simulink library "RfftLib"  (R2022b)
settings: Solver=VariableStepAuto  StartTime=0.0  StopTime=10.0  RelTol=1e-3
libraries: HandyTextFile x7, ITC x2, $bdroot x2
settings Model: Creator=ud1041536  LastModifiedBy=fz1054048
settings SolverCC: AlgebraicLoopSolver=TrustRegion
settings DebuggingCC: UnconnectedInputMsg=warning  UnconnectedOutputMsg=warning  UnconnectedLineMsg=warning  SFMachineParentedDataDiag=warning  ArithmeticOperatorsInVariantConditions=warning
settings ModelReferenceCC: EnableRefExpFcnMdlSchedulingChecks=on
settings SFSimCC: CustomCodeUndefinedFunction=UseInterfaceOnly
settings RTWCC: DLArmComputeVersion=19.05

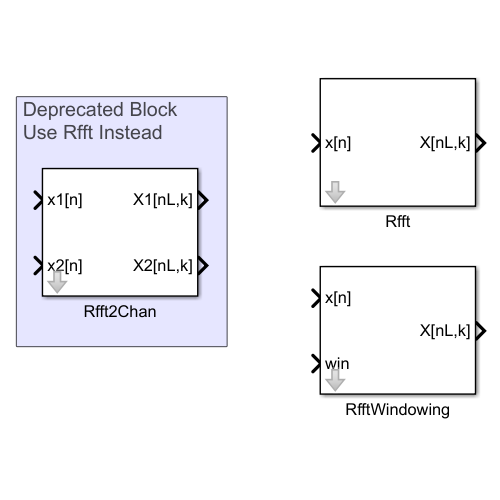
[thumbnail: Simulink's stored preview of the top-level diagram]
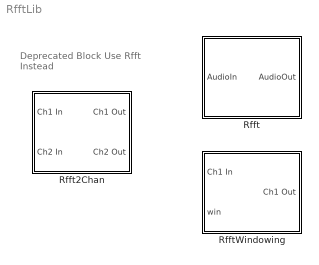
== system RfftLib ==
  note: Deprecated Block
      | Use Rfft Instead
  Rfft : Subsystem  Description=This block computes the Fourier Transform using an optimized FFT for real 2-channel input.  mask(Blocklib Rfft){Config=[]}
      mask prompts: Config "RfftConfig"
      mask help:
      | See 'Help' or run
      | >> help RfftConfig
      mask init:
      | blkh=gcbh;
      | Config=BTConfig.Assert(blkh,Config);
      | 
      | Config.Validate();
      | Config.DoMaskInit(blkh);
      mask Help: eval('help RfftConfig')
      mask Display:
      | port_label('input',1,'x[n]')
      | port_label('output',1,'X[nL,k]')
  Rfft2Chan : Subsystem  Description=This block computes the Fourier Transform using an optimized FFT for real 2-channel input.  mask(Blocklib Rfft2Chan){Config=[]}
      mask prompts: Config "Rfft2ChanConfig"
      mask help:
      | See 'Help' or run
      | >> help Rfft2ChanConfig
      mask init:
      | blkh=gcbh;
      | 
      | Config=BTConfig.Assert(blkh,Config);
      | 
      | Config.Validate();
      | Config.DoMaskInit(blkh);
      mask Help: eval('help Rfft2ChanConfig')
      mask Display:
      | port_label('input',1,'x1[n]')
      | port_label('input',2,'x2[n]')
      | port_label('output',1,'X1[nL,k]')
      | port_label('output',2,'X2[nL,k]')
  RfftWindowing : Subsystem  Description=This block computes the Fourier Transform using an optimized FFT for real 2-channel input.  mask(Blocklib RfftWindowing){Config=[]}
      mask prompts: Config "RfftWindowingConfig"
      mask help:
      | See 'Help' or run
      | >> help RfftWindowingConfig
      mask init:
      | blkh=gcbh;
      | Config=BTConfig.Assert(blkh,Config);
      | 
      | Config.Validate();
      | Config.DoMaskInit(blkh);
      mask Help: eval('help RfftWindowingConfig')
      mask Display:
      | port_label('input',1,'x[n]')
      | port_label('input',2,'win')
      | port_label('output',1,'X[nL,k]')

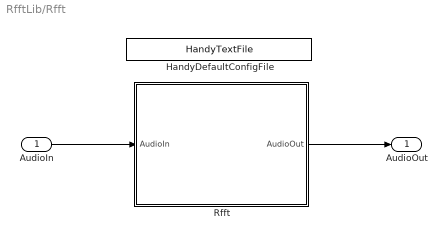
== system RfftLib/Rfft ==
  AudioIn : Inport
  HandyDefaultConfigFile : HandyTextFile/HandyTextFile  TemplateSource=Config  FileSuffix=Init  OpenDialogOnLoad=off  UseThisBlockName=off  AddGrandParentNamePrefix=off  TheDefaultText=|  ShowInLibBrowser=on
      | % $(FILENAME) Setup model parameters for each "Init" callback (e.g. update diagram)
      | sample_rate_in_hertz = 44100;
      | frame_size = 32;
      | sysin_channel_count = 2;
      settings: SourceProductName=Bose Talaria
  Rfft : Subsystem  Variant=on  VariantControl=Choice
  AudioOut : Outport  VectorParamsAs1DForOutWhenUnconnected=off
      settings: SignalType=complex
  wires:
  Rfft/1(AudioOut) -> AudioOut/1
  AudioIn/1 -> Rfft/1(AudioIn)

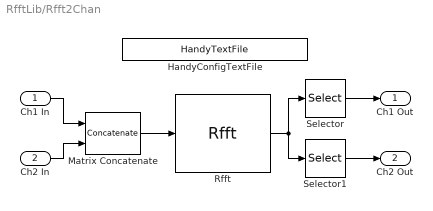
== system RfftLib/Rfft2Chan ==
  Ch1 In : Inport
  Ch2 In : Inport  Port=2
  HandyConfigTextFile : HandyTextFile/HandyTextFile  TemplateSource=Config  FileSuffix=File  OpenDialogOnLoad=off  UseThisBlockName=off  AddGrandParentNamePrefix=off  TheDefaultText=% $(FILENAME) $(PREFIX) $(SUFFIX)  ShowInLibBrowser=on
      settings: SourceProductName=Bose Talaria
  Matrix Concatenate : Concatenate  Mode=Multidimensional array  ConcatenateDimension=2
  Rfft : $bdroot/Rfft  Description=This block computes the Fourier Transform using an optimized FFT for real 2-channel input.  Config=Config
  Selector : Selector  NumberOfDimensions=2  InputPortWidth=3  IndexOptions=Select all,Index vector (dialog)  Indices=[1 3],1  OutputSizes=1,1
  Selector1 : Selector  NumberOfDimensions=2  InputPortWidth=3  IndexOptions=Select all,Index vector (dialog)  Indices=[1 3],2  OutputSizes=1,1
  Ch1 Out : Outport  VectorParamsAs1DForOutWhenUnconnected=off
  Ch2 Out : Outport  Port=2  VectorParamsAs1DForOutWhenUnconnected=off
  wires:
  Ch1 In/1 -> Matrix Concatenate/1
  Ch2 In/1 -> Matrix Concatenate/2
  Matrix Concatenate/1 -> Rfft/1
  Selector/1 -> Ch1 Out/1
  Rfft/1 -> Selector1/1, Selector/1
  Selector1/1 -> Ch2 Out/1

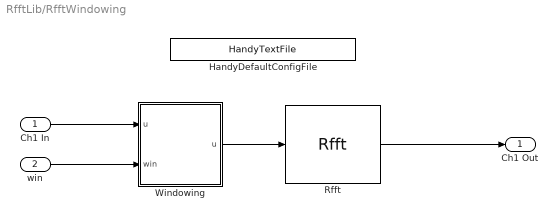
== system RfftLib/RfftWindowing ==
  Ch1 In : Inport
  win : Inport  Port=2
  HandyDefaultConfigFile : HandyTextFile/HandyTextFile  TemplateSource=Config  FileSuffix=Init  OpenDialogOnLoad=off  UseThisBlockName=off  AddGrandParentNamePrefix=off  TheDefaultText=|  ShowInLibBrowser=on
      | % $(FILENAME) Setup model parameters for each "Init" callback (e.g. update diagram)
      | sample_rate_in_hertz = 44100;
      | frame_size = 32;
      | sysin_channel_count = 2;
      settings: SourceProductName=Bose Talaria
  Rfft : $bdroot/Rfft  Description=This block computes the Fourier Transform using an optimized FFT for real 2-channel input.  Config=Config
  Windowing : MATLAB Function  TreatAsAtomicUnit=on
  Ch1 Out : Outport  VectorParamsAs1DForOutWhenUnconnected=off
      settings: SignalType=complex
  wires:
  Rfft/1 -> Ch1 Out/1
  Windowing/1(u) -> Rfft/1
  Ch1 In/1 -> Windowing/1("u ")
  win/1 -> Windowing/2(win)

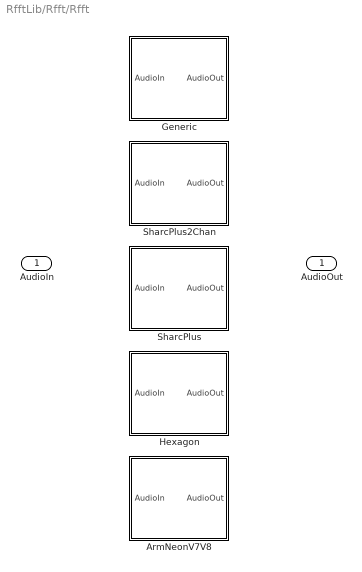
== system RfftLib/Rfft/Rfft ==
  AudioIn : Inport
  ArmNeonV7V8 : Subsystem  VariantControl=(Config.Breed == AsdHwEnum.ArmNeonV7V8)
  Generic : Subsystem  VariantControl=(default)
  Hexagon : Subsystem  VariantControl=(Config.Breed == AsdHwEnum.Hexagon)
  SharcPlus : Subsystem  VariantControl=(Config.Breed == AsdHwEnum.SharcPlus) && (Config.NumChannels ~= 2)
  SharcPlus2Chan : Subsystem  VariantControl=(Config.Breed == AsdHwEnum.SharcPlus) && (Config.NumChannels == 2)
  AudioOut : Outport

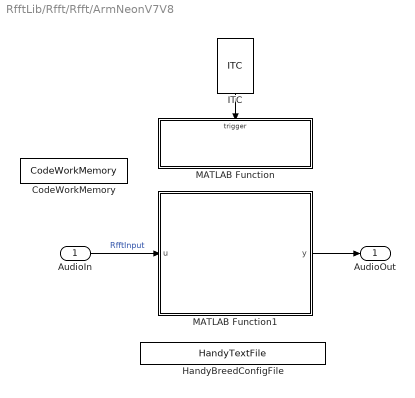
== system RfftLib/Rfft/Rfft/ArmNeonV7V8 ==
  AudioIn : Inport
  CodeWorkMemory : DataStoreMemory  DataStoreName=CodeWorkMemory  WriteAfterWriteMsg=warning  InitialValue=Config.BreedObj.DsmCodeWorkMemoryInitValue  ShowAdditionalParam=off  OutDataTypeStr=uint32
  HandyBreedConfigFile : HandyTextFile/HandyTextFile  TemplateSource=<dialog fields>  FileSuffix=BreedConfig  OpenDialogOnLoad=off  UseThisBlockName=off  AddGrandParentNamePrefix=on  TheDefaultText=|  ShowInLibBrowser=on
      | % $(FILENAME) Setup model parameters for each "Init" callback (e.g. update diagram)
      | sample_rate_in_hertz = 44100;
      | frame_size = 32;
      | sysin_channel_count = 2;
      settings: SourceProductName=Bose Talaria
  ITC : ITC/ITC
      settings: SourceProductName=Bose Talaria
  MATLAB Function : MATLAB Function  TreatAsAtomicUnit=on  mask{fftSize=Config.FftSize}
  MATLAB Function1 : MATLAB Function  TreatAsAtomicUnit=on  mask{fftSize=Config.FftSize}
  AudioOut : Outport  VectorParamsAs1DForOutWhenUnconnected=off
  wires:
  ITC/1 -> MATLAB Function/Trigger
  AudioIn/1 -> MATLAB Function1/1(u)  "RfftInput"
  MATLAB Function1/1(y) -> AudioOut/1

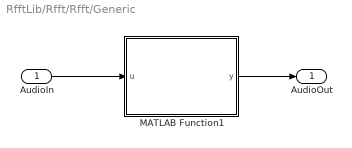
== system RfftLib/Rfft/Rfft/Generic ==
  AudioIn : Inport
  MATLAB Function1 : MATLAB Function  TreatAsAtomicUnit=on  mask{fftSize=Config.FftSize}
  AudioOut : Outport  VectorParamsAs1DForOutWhenUnconnected=off
  wires:
  AudioIn/1 -> MATLAB Function1/1(u)
  MATLAB Function1/1(y) -> AudioOut/1

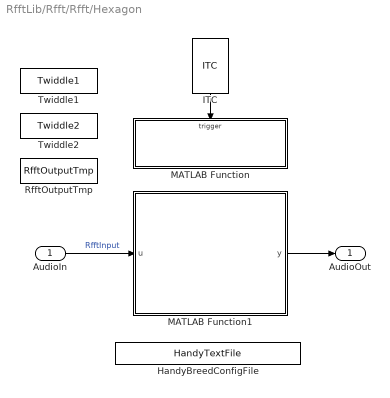
== system RfftLib/Rfft/Rfft/Hexagon ==
  AudioIn : Inport
  HandyBreedConfigFile : HandyTextFile/HandyTextFile  TemplateSource=<dialog fields>  FileSuffix=BreedConfig  OpenDialogOnLoad=off  UseThisBlockName=off  AddGrandParentNamePrefix=on  TheDefaultText=|  ShowInLibBrowser=on
      | % $(FILENAME) Setup model parameters for each "Init" callback (e.g. update diagram)
      | sample_rate_in_hertz = 44100;
      | frame_size = 32;
      | sysin_channel_count = 2;
      settings: SourceProductName=Bose Talaria
  ITC : ITC/ITC
      settings: SourceProductName=Bose Talaria
  MATLAB Function : MATLAB Function  TreatAsAtomicUnit=on  mask{fftSize=Config.FftSize}
  MATLAB Function1 : MATLAB Function  TreatAsAtomicUnit=on  mask{fftSize=Config.FftSize}
  RfftOutputTmp : DataStoreMemory  DataStoreName=RfftOutputTmp  WriteAfterWriteMsg=warning  InitialValue=Config.BreedObj.DsmRfftOutputTmpInitValue  ShowAdditionalParam=off  OutDataTypeStr=single
      settings: SignalType=complex
  Twiddle1 : DataStoreMemory  DataStoreName=Twiddle1  WriteAfterWriteMsg=warning  InitialValue=Config.BreedObj.DsmTwiddle1InitValue  ShowAdditionalParam=off  OutDataTypeStr=single
      settings: SignalType=complex
  Twiddle2 : DataStoreMemory  DataStoreName=Twiddle2  WriteAfterWriteMsg=warning  InitialValue=Config.BreedObj.DsmTwiddle2InitValue  ShowAdditionalParam=off  OutDataTypeStr=single
      settings: SignalType=complex
  AudioOut : Outport  VectorParamsAs1DForOutWhenUnconnected=off
  wires:
  ITC/1 -> MATLAB Function/Trigger
  AudioIn/1 -> MATLAB Function1/1(u)  "RfftInput"
  MATLAB Function1/1(y) -> AudioOut/1

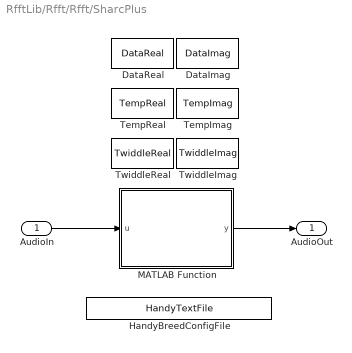
== system RfftLib/Rfft/Rfft/SharcPlus ==
  AudioIn : Inport
  DataImag : DataStoreMemory  DataStoreName=DataImag  ReadBeforeWriteMsg=warning  WriteAfterWriteMsg=warning  WriteAfterReadMsg=warning  InitialValue=Config.BreedObj.DsmDataImagInitValue  ShowAdditionalParam=off  OutDataTypeStr=single
  DataReal : DataStoreMemory  DataStoreName=DataReal  ReadBeforeWriteMsg=warning  WriteAfterWriteMsg=warning  WriteAfterReadMsg=warning  InitialValue=Config.BreedObj.DsmDataRealInitValue  ShowAdditionalParam=off  OutDataTypeStr=single
  HandyBreedConfigFile : HandyTextFile/HandyTextFile  TemplateSource=<dialog fields>  FileSuffix=BreedConfig  OpenDialogOnLoad=off  UseThisBlockName=off  AddGrandParentNamePrefix=on  TheDefaultText=|  ShowInLibBrowser=on
      | % $(FILENAME) Setup model parameters for each "Init" callback (e.g. update diagram)
      | sample_rate_in_hertz = 44100;
      | frame_size = 32;
      | sysin_channel_count = 2;
      settings: SourceProductName=Bose Talaria
  MATLAB Function : MATLAB Function  TreatAsAtomicUnit=on  mask{fftSize=Config.FftSize}
  TempImag : DataStoreMemory  DataStoreName=TempImag  ReadBeforeWriteMsg=warning  WriteAfterWriteMsg=warning  WriteAfterReadMsg=warning  InitialValue=Config.BreedObj.DsmTempImagInitValue  ShowAdditionalParam=off  OutDataTypeStr=single
  TempReal : DataStoreMemory  DataStoreName=TempReal  ReadBeforeWriteMsg=warning  WriteAfterWriteMsg=warning  WriteAfterReadMsg=warning  InitialValue=Config.BreedObj.DsmTempRealInitValue  ShowAdditionalParam=off  OutDataTypeStr=single
  TwiddleImag : DataStoreMemory  DataStoreName=TwiddleImag  ReadBeforeWriteMsg=warning  WriteAfterWriteMsg=warning  WriteAfterReadMsg=warning  InitialValue=Config.BreedObj.DsmTwiddleImagInitValue  ShowAdditionalParam=off  OutDataTypeStr=uint32
  TwiddleReal : DataStoreMemory  DataStoreName=TwiddleReal  ReadBeforeWriteMsg=warning  WriteAfterWriteMsg=warning  WriteAfterReadMsg=warning  InitialValue=Config.BreedObj.DsmTwiddleRealInitValue  ShowAdditionalParam=off  OutDataTypeStr=uint32
  AudioOut : Outport  VectorParamsAs1DForOutWhenUnconnected=off
  wires:
  MATLAB Function/1(y) -> AudioOut/1
  AudioIn/1 -> MATLAB Function/1(u)

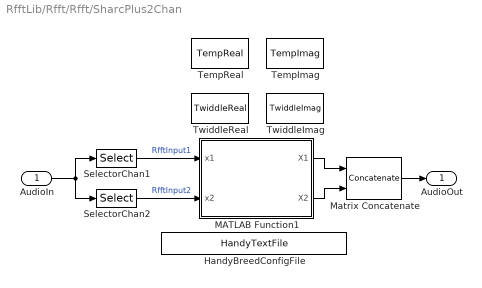
== system RfftLib/Rfft/Rfft/SharcPlus2Chan ==
  AudioIn : Inport
  HandyBreedConfigFile : HandyTextFile/HandyTextFile  TemplateSource=<dialog fields>  FileSuffix=BreedConfig  OpenDialogOnLoad=off  UseThisBlockName=off  AddGrandParentNamePrefix=on  TheDefaultText=|  ShowInLibBrowser=on
      | % $(FILENAME) Setup model parameters for each "Init" callback (e.g. update diagram)
      | sample_rate_in_hertz = 44100;
      | frame_size = 32;
      | sysin_channel_count = 2;
      settings: SourceProductName=Bose Talaria
  MATLAB Function1 : MATLAB Function  TreatAsAtomicUnit=on  mask{fftSize=Config.FftSize}
  Matrix Concatenate : Concatenate  Mode=Multidimensional array  ConcatenateDimension=2
  SelectorChan1 : Selector  NumberOfDimensions=2  InputPortWidth=3  IndexOptions=Select all,Index vector (dialog)  Indices=[1 3],1  OutputSizes=1,1
  SelectorChan2 : Selector  NumberOfDimensions=2  InputPortWidth=3  IndexOptions=Select all,Index vector (dialog)  Indices=[1 3],2  OutputSizes=1,1
  TempImag : DataStoreMemory  DataStoreName=TempImag  ReadBeforeWriteMsg=warning  WriteAfterWriteMsg=warning  WriteAfterReadMsg=warning  InitialValue=Config.BreedObj.DsmTempImagInitValue  ShowAdditionalParam=off  OutDataTypeStr=single
  TempReal : DataStoreMemory  DataStoreName=TempReal  ReadBeforeWriteMsg=warning  WriteAfterWriteMsg=warning  WriteAfterReadMsg=warning  InitialValue=Config.BreedObj.DsmTempRealInitValue  ShowAdditionalParam=off  OutDataTypeStr=single
  TwiddleImag : DataStoreMemory  DataStoreName=TwiddleImag  ReadBeforeWriteMsg=warning  WriteAfterWriteMsg=warning  WriteAfterReadMsg=warning  InitialValue=Config.BreedObj.DsmTwiddleImagInitValue  ShowAdditionalParam=off  OutDataTypeStr=uint32
  TwiddleReal : DataStoreMemory  DataStoreName=TwiddleReal  ReadBeforeWriteMsg=warning  WriteAfterWriteMsg=warning  WriteAfterReadMsg=warning  InitialValue=Config.BreedObj.DsmTwiddleRealInitValue  ShowAdditionalParam=off  OutDataTypeStr=uint32
  AudioOut : Outport  VectorParamsAs1DForOutWhenUnconnected=off
  wires:
  MATLAB Function1/2(X2) -> Matrix Concatenate/2
  MATLAB Function1/1(X1) -> Matrix Concatenate/1
  AudioIn/1 -> SelectorChan2/1, SelectorChan1/1
  SelectorChan1/1 -> MATLAB Function1/1(x1)  "RfftInput1"
  SelectorChan2/1 -> MATLAB Function1/2(x2)  "RfftInput2"
  Matrix Concatenate/1 -> AudioOut/1

== matlab function RfftLib/Rfft/Rfft/SharcPlus2Chan/MATLAB Function1 ==
  data: x1 input; x2 input; X1 output; fftSize parameter; X2 output; TempReal data_store_memory; TempImag data_store_memory; TwiddleReal data_store_memory; TwiddleImag data_store_memory
function [X1, X2] = Rfft(x1, x2, fftSize)   

global TempReal
global TempImag
global TwiddleReal
global TwiddleImag

% Nullcopy copies type, size, and complexity to output
X1 = coder.nullcopy(complex(single(zeros((fftSize/2) + 1, 1))));
X2 = coder.nullcopy(complex(single(zeros((fftSize/2) + 1, 1))));

% Set correct data types
fftSize = uint32(fftSize);

% Simulation
if(coder.target('MATLAB') || coder.target('Sfun')) 
    [X1, X2] = Rfft2ChanProcessSim(x1, x2, fftSize);

% Code generation
else
    % GUL
    % Set the twiddle pointers to correct twiddle table
    % The pointers are of type uint32 here and will be casted to float* 
    % in the code-replaced function. The twiddle tables are declared in 
    % a separate file and will be pulled in through CRL.
    if fftSize == 256
        coder.ceval('set_twiddle_256', coder.wref(TwiddleReal), coder.wref(TwiddleImag));
    else
        coder.ceval('set_twiddle_128', coder.wref(TwiddleReal), coder.wref(TwiddleImag));
    end
    [X1, X2] = rfft_inplace_process(x1, x2, TempReal, TempImag, ...
        TwiddleReal, TwiddleImag, fftSize);

end
    
end

%% CRL function for code generation SHARC+
function [y1, y2] = rfft_inplace_process(u1, u2, temp_r, temp_i, ...
    twiddle_r, twiddle_i, fft_size)
% If target == codegen, error out if no CRL found
coder.replace('-errorifnoreplacement');

half_spectrum_size = (fft_size/2) + 1;
y1 = complex(single(zeros(half_spectrum_size, 1)));
y2 = complex(single(zeros(half_spectrum_size, 1)));
end

== matlab function RfftLib/Rfft/Rfft/ArmNeonV7V8/MATLAB Function ==
  data: fftSize parameter; CodeWorkMemory data_store_memory
  events: trigger input FUNCTION_CALL_EVENT
function RfftInit(fftSize)
% Initializes the Twiddle factors used for RFFT computation

global CodeWorkMemory;

if ~(coder.target('MATLAB') || coder.target('Sfun')) 
    y = rfft_armv7v8_init(uint32(fftSize), uint32(CodeWorkMemory));    
    % NOTE: The CRL mechanism requires an output for the function call,
    % and appears to be optimized out if that return value isn't used. 
    % This is a dummy operation to make sure CRL ends up in generated code    
    CodeWorkMemory(1) = y;
end
end


function y = rfft_armv7v8_init(fftSize, workMemory)
% If target == codegen, error out if no CRL found
coder.replace('-errorifnoreplacement');
% No init simulation code, but need to do something to ensure CRL does not
% get optimized out
y = uint32(workMemory(1)) + fftSize;
end

== matlab function RfftLib/Rfft/Rfft/ArmNeonV7V8/MATLAB Function1 ==
  data: u input; y output; fftSize parameter; CodeWorkMemory data_store_memory
function y = Rfft(u, fftSize)   
% Computes the Real FFT of a Multi-Channel Signal. 
% During Code Generation, ArmNeonV7V8 rfft crl function is used.
% Inputs:
%     u - purely real signal. 
%         size = [fftSize, numChannels]
%     fftSize - size of each input channel. Also the size of FFT
% Outputs:
%     y - fftSize/2 + 1 unique FFT coefficients of each channel of u.
%         size = [fftSize/2 + 1, numChannels]
% -------------------------------------------------------------------------

global CodeWorkMemory

NumChannels = size(u, 2);
HalfSpectrumSize = (fftSize/2) + 1;

% Nullcopy copies type, size, and complexity of input to output
y = coder.nullcopy(complex(single(zeros(HalfSpectrumSize, NumChannels))));

% Simulation
if(coder.target('MATLAB') || coder.target('Sfun')) 
    y = RfftProcessSim(u, fftSize);
% Code generation
else
    y = complex(rfft_armv7v8_process(single(u), uint32(fftSize), CodeWorkMemory, uint32(NumChannels)));
end

end

%% CRL function for code generation ARM
function y = rfft_armv7v8_process(u, fftSize, workMemory, NumChannels)
% If target == codegen, error out if no CRL found
coder.replace('-errorifnoreplacement');

half_spectrum_size = (fftSize/2) + 1;
y = complex(single(zeros(half_spectrum_size, NumChannels)));
end

== matlab function RfftLib/Rfft/Rfft/Generic/MATLAB Function1 ==
  data: u input; y output; fftSize parameter
function y = Rfft(u, fftSize)

y = RfftProcessSim(u, fftSize);

end

== matlab function RfftLib/RfftWindowing/Windowing ==
  data: u input; win input; u output
function u = fcn(u, win)

% Get sizes
[~, numChannels] = size(u);

% Loop since array-vector multiply operation doesn't work here
% Input/Output have the same variable name for in-place processing
for i = 1:numChannels
    u(:, i) = u(:,i) .* win;
end

end

== matlab function RfftLib/Rfft/Rfft/Hexagon/MATLAB Function ==
  data: fftSize parameter; Twiddle1 data_store_memory; Twiddle2 data_store_memory
  events: trigger input FUNCTION_CALL_EVENT
function RfftInit(fftSize)
% Initializes the Twiddle factors used for RFFT computation

global Twiddle1;
global Twiddle2;

% Intialize Twiddle Factors
[Twiddle1, Twiddle2] = rfft_init(int32(fftSize));

end

function [Twiddle1, Twiddle2] = rfft_init(fftSize)
% Twiddle1: Twiddle factor for N/2-point complex FFT
% Twiddle2: Twiddle factors for last stage
% If target == codegen, error out if no CRL found
coder.replace('-errorifnoreplacement');
Twiddle1 = single(complex(zeros(3*fftSize/8,1)));
Twiddle2 = single(complex(zeros(fftSize/2,1)));

end

== matlab function RfftLib/Rfft/Rfft/Hexagon/MATLAB Function1 ==
  data: u input; y output; fftSize parameter; RfftOutputTmp data_store_memory; Twiddle1 data_store_memory; Twiddle2 data_store_memory
function y = Rfft(u, fftSize)   
% Computes the Real FFT of a Multi-Channel Signal. 
% During Code Generation, hexagon rfft crl function is used.
% Inputs:
%     u - purely real signal. 
%         size = [fftSize, numChannels]
%     fftSize - size of each input channel. Also the size of FFT
% Outputs:
%     y - fftSize/2 + 1 unique FFT coefficients of each channel of u.
%         size = [fftSize/2 + 1, numChannels]
% -------------------------------------------------------------------------

global RfftOutputTmp;
global Twiddle1;
global Twiddle2;

numChannels = size(u, 2);
spectrumSize = (fftSize/2) + 1;

% Nullcopy copies type, size, and complexity of input to output
y = coder.nullcopy(complex(single(zeros(spectrumSize, numChannels))));

% Simulation
if(coder.target('MATLAB') || coder.target('Sfun')) 
    y = RfftProcessSim(u, fftSize);
% Code generation
else
    y = rfft_process(single(u), Twiddle1, Twiddle2, RfftOutputTmp, int32(fftSize), int32(numChannels));
end

end

%% CRL function for code generation HEXAGON
function y = rfft_process(u, twiddle1, twiddle2, outputTmp, fftSize, numChannels);
% If target == codegen, error out if no CRL found
coder.replace('-errorifnoreplacement');

half_spectrum_size = (fftSize/2) + 1;
y = complex(single(zeros(half_spectrum_size, numChannels)));

end

== matlab function RfftLib/Rfft/Rfft/SharcPlus/MATLAB Function ==
  data: u input; y output; fftSize parameter; DataReal data_store_memory; DataImag data_store_memory; TempReal data_store_memory; TempImag data_store_memory; TwiddleReal data_store_memory; TwiddleImag data_store_memory
function y = Rfft(u, fftSize)   

global DataReal
global DataImag
global TempReal
global TempImag
global TwiddleReal
global TwiddleImag

[~, numChannels] = size(u);
spectrumSize = (fftSize/2) + 1;

% Nullcopy copies type, size, and complexity of input to output
y = coder.nullcopy(complex(single(zeros(spectrumSize, numChannels))));

% Set correct data types
fftSize = uint32(fftSize);
numChannels = uint32(numChannels);

% Simulation
if(coder.target('MATLAB') || coder.target('Sfun')) 
    y = RfftProcessSim(u, fftSize);
    
% Code generation
else
    % Set the twiddle pointers to correct twiddle table
    % The pointers are of type uint32 here and will be casted to float* 
    % in the code-replaced function. The twiddle tables are declared in 
    % a separate file and will be pulled in through CRL.
    if fftSize == 256
        coder.ceval('set_twiddle_256', coder.wref(TwiddleReal), coder.wref(TwiddleImag));
    else
        coder.ceval('set_twiddle_128', coder.wref(TwiddleReal), coder.wref(TwiddleImag));
    end
    y = rfft_process(u, DataReal, DataImag, TempReal, TempImag, ...
        TwiddleReal, TwiddleImag, fftSize, numChannels);

end

end

%% CRL function for code generation
function y = rfft_process(u, data_r, data_i, temp_r, temp_i, ...
    twiddle_r, twiddle_i, fft_size, num_channels)
% If target == codegen, error out if no CRL found
coder.replace('-errorifnoreplacement');

y = RfftProcessSim(u, fft_size);
end
